simulink model "sim_ab"  (R2017b)
settings: Solver=VariableStepAuto  StartTime=0.0  StopTime=200.0  RelTol=1e-3
settings Model: Creator=piopi  LastModifiedBy=piopi

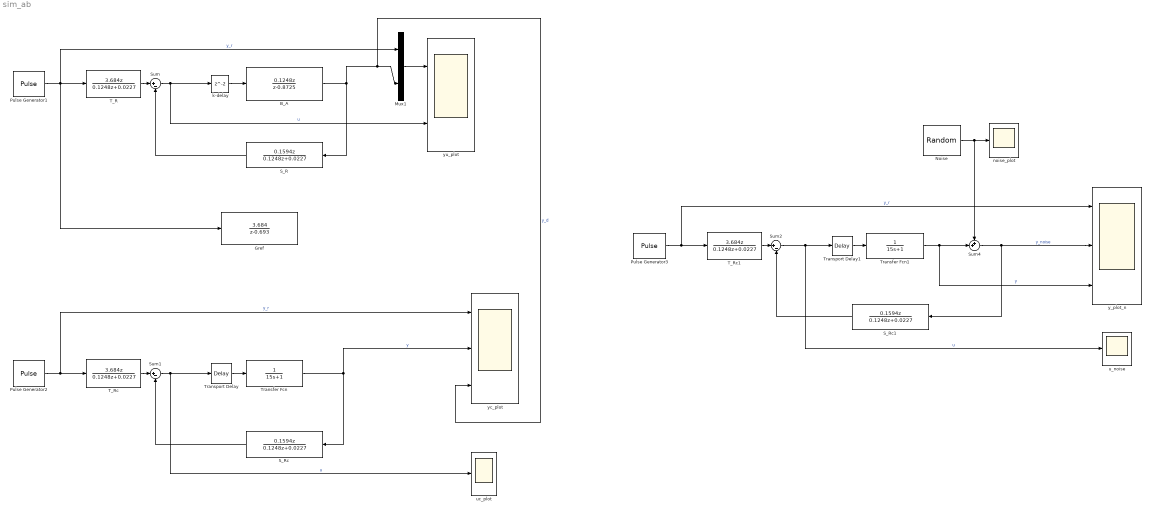
== system sim_ab ==
  B_A : DiscreteTransferFcn  Numerator=[0.1248 0]  Denominator=[1 -0.8725]  SampleTime=2
  Gref : DiscreteTransferFcn  Numerator=[3.684]  Denominator=[1, -0.693]  SampleTime=2
  Mux1 : Mux  Inputs=2
  Noise : RandomNumber  Variance=0.1  SampleTime=0.1
  Pulse Generator1 : DiscretePulseGenerator  PulseType=Time based  Period=240  PulseWidth=50
  Pulse Generator2 : DiscretePulseGenerator  PulseType=Time based  Period=240  PulseWidth=50
  Pulse Generator3 : DiscretePulseGenerator  PulseType=Time based  Period=240  PulseWidth=50
  S_R : DiscreteTransferFcn  Numerator=[0.1594 0]  Denominator=[0.1248, 0.0227]  SampleTime=2
  S_Rc : DiscreteTransferFcn  Numerator=[0.1594 0]  Denominator=[0.1248, 0.0227]  SampleTime=2
  S_Rc1 : DiscreteTransferFcn  Numerator=[0.1594 0]  Denominator=[0.1248, 0.0227]  SampleTime=2
  Sum : Sum  Inputs=|+-
  Sum1 : Sum  Inputs=|+-
  Sum2 : Sum  Inputs=|+-
  Sum4 : Sum  Inputs=++|
  T_R : DiscreteTransferFcn  Numerator=[3.684 0]  Denominator=[0.1248, 0.0227]  SampleTime=2
  T_Rc : DiscreteTransferFcn  Numerator=[3.684 0]  Denominator=[0.1248, 0.0227]  SampleTime=2
  T_Rc1 : DiscreteTransferFcn  Numerator=[3.684 0]  Denominator=[0.1248, 0.0227]  SampleTime=2
  Transfer Fcn : TransferFcn  Denominator=[15 1]
  Transfer Fcn1 : TransferFcn  Denominator=[15 1]
  Transport Delay : TransportDelay  DelayTime=2
  Transport Delay1 : TransportDelay  DelayTime=2
  k-delay : Delay  SampleTime=2
  noise_plot : Scope
  u_noise : Scope
  uc_plot : Scope
  y_plot_n : Scope  NumInputPorts=3
  yc_plot : Scope  NumInputPorts=3
  yu_plot : Scope  NumInputPorts=2
  wires:
  Sum/1 -> k-delay/1, yu_plot/2  "u"
  Pulse Generator1/1 -> Gref/1, Mux1/1, T_R/1  "y_r"
  B_A/1 -> S_R/1, yc_plot/3, Mux1/2  "y_d"
  Mux1/1 -> yu_plot/1
  T_R/1 -> Sum/1
  S_R/1 -> Sum/2
  k-delay/1 -> B_A/1
  T_Rc/1 -> Sum1/1
  Sum1/1 -> uc_plot/1, Transport Delay/1  "u"
  Pulse Generator2/1 -> yc_plot/1, T_Rc/1  "y_r"
  S_Rc/1 -> Sum1/2
  Transfer Fcn/1 -> yc_plot/2, S_Rc/1  "y"
  Transport Delay/1 -> Transfer Fcn/1
  T_Rc1/1 -> Sum2/1
  Sum2/1 -> u_noise/1, Transport Delay1/1  "u"
  Pulse Generator3/1 -> y_plot_n/1, T_Rc1/1  "y_r"
  S_Rc1/1 -> Sum2/2
  Transport Delay1/1 -> Transfer Fcn1/1
  Noise/1 -> noise_plot/1, Sum4/1
  Transfer Fcn1/1 -> y_plot_n/3, Sum4/2  "y"
  Sum4/1 -> y_plot_n/2, S_Rc1/1  "y_noise"
